simulink model "plant_control"  (R2017a)
settings: Solver=VariableStepAuto  StartTime=0.0  StopTime=10.0  RelTol=1e-3
values from neighbouring files (symbols this model uses):
  x = x_1 + (dt/6)*(k1 + 2*k2 + 2*k3 + k4)    [my_ode45.m]
  x0 = 100    [validate_model.m]
undefined symbols (not defined in the file or in its folder): controlfun, plantfun
settings Model: Creator=bruno  LastModifiedBy=bruno

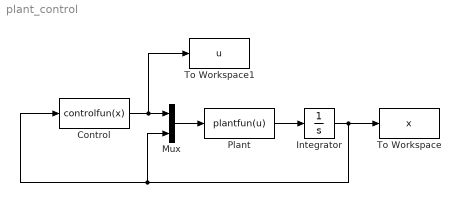
== system plant_control ==
  "Control " : MATLABFcn  MATLABFcn=controlfun(x)  OutputSignalType=real
  Integrator : Integrator  InitialCondition=x0
  Mux : Mux  Inputs=2
  Plant : MATLABFcn  MATLABFcn=plantfun(u)  OutputSignalType=real
  To Workspace : ToWorkspace  VariableName=x  SaveFormat=Timeseries  SampleTime=-1
  To Workspace1 : ToWorkspace  VariableName=u  SaveFormat=Timeseries  SampleTime=-1
  wires:
  Plant/1 -> Integrator/1
  Integrator/1 -> To Workspace/1, "Control "/1, Mux/2
  Mux/1 -> Plant/1
  "Control "/1 -> To Workspace1/1, Mux/1
